simulink library "GRC_Lib"  (R2017b)
settings: Solver=VariableStepAuto  StartTime=0.0  StopTime=10.0  RelTol=1e-3  EnableMultiTasking=on
StartFcn:
  | set_param('AdvancedOperations','ZoomFactor','100');
undefined symbols (not defined in the file): Test
libraries: GRC_Lib x203, simulink x1
(part 3 of 4)

== system GRC_Lib/Routing ==
  Selector : Subsystem  TreatAsAtomicUnit=on  mask{IpDT=double, SizeUMsk=6}
      mask prompts: IpDT "Input U Data Type"; SizeUMsk "Input Port Size (Min 1)"
      mask init:
      | if isequal(str2num(get_param(gcb,'SizeUMsk')),[])
      |    if SizeUMsk<1
      |        error('*** ERROR ***    Input Port Size must be integer and >=1.');
      |    elseif SizeUMsk<256
      |        SizeU = SizeUMsk; 
      |        set_param([gcb '/Constant'],'OutDataTypeStr','uint8');
      |        set_param([gcb '/Constant'],'Value', mat2str(SizeUMsk-1));
      |    elseif SizeUMsk<=65535 
      |        SizeU = SizeUMsk; 
      |        set_param([gcb '/Constant'],'OutDataTypeStr','uint16');
      |        set_param([gcb '/Constant'],'Value', mat2str(SizeUMsk-1));
      |    else
      |        SizeU = SizeUMsk;
      |        set_param([gcb '/Constant'],'OutDataTypeStr','uint32');
      |        set_param([gcb '/Constant'],'Value', mat2str(SizeUMsk-1));
      |    end
      | else
      |     SizeNmbr = str2num(get_param(gcb,'SizeUMsk'));
      |    if SizeNmbr<1
      |        error('*** ERROR ***    Input Port Size must be integer and >=1.');
      |    elseif SizeNmbr<256
      |        SizeU = SizeUMsk;
      |        set_param([gcb '/Constant'],'OutDataTypeStr','uint8');
      |        set_param([gcb '/Constant'],'Value', mat2str(SizeNmbr-1));
      |    elseif SizeNmbr<=65535 
      |        SizeU = SizeNmbr;
      |        set_param([gcb '/Constant'],'OutDataTypeStr','uint16');
      |        set_param([gcb '/Constant'],'Value', mat2str(SizeNmbr-1));
      |    else
      |        SizeU = SizeNmbr;
      |        set_param([gcb '/Constant'],'OutDataTypeStr','uint32');
      |        set_param([gcb '/Constant'],'Value', mat2str(SizeNmbr-1));
      |    end 
      | end
      | 
      | DTStry = get_param(gcb,'IpDT');
      | try
      |     if isequal(DTStry,'boolean')
      |         FColor = '[0.901961, 0.313725, 0.078431]'; 
      |     elseif isequal(DTStry,'double')||isequal(DTStry,'single')
      |         FColor = '[0.313725, 0.117647, 0.352941]';  
      |     else
      |         FColor = '[0.196078, 0.549020, 0.549020]';
      |     end        
      | catch
      | end
      | set_param([gcb '/Y'],'ForegroundColor',FColor);
      | set_param(gcb,'ForegroundColor',FColor);
      settings: AttributesFormatString=SizeU = %<SizeUMsk>
      mask Callback SizeUMsk:
      | % if isequal(str2num(get_param(gcb,'SizeUMsk')),[])
      | %    if SizeUMsk<1
      | %        error('*** ERROR ***    Input Port Size must be integer and >=1.');
      | %    else
      | %    end
      | % else
      | %    if str2num(get_param(gcb,'SizeUMsk'))<1
      | %        error('*** ERROR ***    Input Port Size must be integer and >=1.');
      | %    else
      | %    end
      | % end
      mask Display:
      | % color('blue');
      | % disp('\bfSlctr','texmode','on');
      | image(imread('Selector.jpg'),[0.3,0.4,0.55,0.8]);
  Vbi_OilTempSensor : Subsystem  TreatAsAtomicUnit=on  mask(MessurementVaraibale){VariableName=Vbi_OilTempSensor, VariableType=Inherit: auto, S_Min=0, S_Max=100}
      mask prompts: VariableName "SignalName"; VariableType "VarableType"; S_Min "Min"; S_Max "Max"
      mask help: messurement Variable
      mask init:
      | hld = get_param([gcb '/In1'],'Object');
      | set(hld,'OutDataTypeStr',get_param(gcb,'VariableType'));
      | set(hld,'OutMin',get_param(gcb,'S_Min'));
      | set(hld,'OutMax',get_param(gcb,'S_Max'));
      | 
      | p_in1 =get_param([gcb '/In1'],'PortHandles');
      | hl_line = get_param(p_in1.Outport,'line');
      | set(hl_line,'Name',get_param(gcb,'VariableName'));
      | set(hl_line,'SignalObjectPackage','AUTOSAR4');
      | set(hl_line,'StorageClass','SimulinkGlobal');
      | 
      | DTStry = get_param(gcb,'VariableType');
      | try
      |     if isequal(DTStry,'boolean')
      |         FColor = '[0.901961, 0.313725, 0.078431]'; 
      |     elseif isequal(DTStry,'double')||isequal(DTStry,'single')
      |         FColor = '[0.313725, 0.117647, 0.352941]';  
      |     else
      |         FColor = '[0.196078, 0.549020, 0.549020]';
      |     end        
      | catch
      | end
      | set_param([gcb '/Out1'],'ForegroundColor',FColor);
      | set_param(gcb,'ForegroundColor',FColor);
      settings: RTWSystemCode=Inline
      mask Display:
      | %plot([0 .78 1 .78 0 0],[0 0 0.5 1 1 0]);
      | %plot([.78 .78],[0 1]);
      | %patch([0 .12 .12 0 0],[0 0 1 1 0],[0 0 0]);
      | color('black');
      | msk_block_name = get_param(gcb,'VariableName');
      | set_param(gcb,'Name',msk_block_name);
      | disp(get_param(gcb,'VariableName'));
      | %mp_in1 = find_system(gcb,'FindAll','on','type','line','name','label');
      | %mp_obj = get_param(mp_in1,'Object');
      | %set(mp_obj,'name',msk_block_name);
      | %set(mp_obj,'RTWStorageClass','SimulinkGloable');

== system GRC_Lib/SignalAttributes ==
  DTC : Subsystem  mask{OpDT=double}
      mask prompts: OpDT "Output Data Type"
      mask init:
      | set_param([gcb '/DTC'],'OutDataTypeStr',OpDT);
      | % set_param([gcb '/Odt'],'OutDataTypeStr',OpDT);
      | 
      | DTStry = get_param([gcb '/DTC'],'OutDataTypeStr');
      | try
      |     if isequal(DTStry,'boolean')
      |         FColor = '[0.901961, 0.313725, 0.078431]'; 
      |     elseif isequal(DTStry,'double')||isequal(DTStry,'single')
      |         FColor = '[0.313725, 0.117647, 0.352941]';  
      |     else
      |         FColor = '[0.196078, 0.549020, 0.549020]';
      |     end        
      | catch
      | end
      | set_param([gcb '/Odt'],'ForegroundColor',FColor);
      | set_param(gcb,'ForegroundColor',FColor);
      mask Display:
      | color('green');
      | disp(get_param(gcb,'OpDT'),'texmode','on');

== system GRC_Lib/SignalSwitch ==
  SWT2 : Subsystem  mask{OpDT=double}
      mask prompts: OpDT "Output Data Type"
      mask init:
      | DTStr = get_param(gcb,'OpDT');
      | try
      |     if isequal(DTStr,'boolean')
      |         FColor = '[0.901961, 0.313725, 0.078431]'; 
      |     elseif isequal(DTStr,'double')||isequal(DTStr,'single')
      |         FColor = '[0.313725, 0.117647, 0.352941]';  
      |     else
      |         FColor = '[0.196078, 0.549020, 0.549020]';
      |     end
      | catch
      | end
      | set_param([gcb '/T'],'ForegroundColor',FColor);
      | set_param([gcb '/F'],'ForegroundColor',FColor);
      | set_param([gcb '/y'],'ForegroundColor',FColor);
      mask Display:
      | % image('SwitchNN2.jpg');
      | image(imread('SWT2.jpg'),[0.25,0.15,0.55,0.85]);
  SWT3 : Subsystem  TreatAsAtomicUnit=on
      mask help:
      | if Rst = 1
      |    y = RstV;
      | else
      |     if E = 1
      |        y = u;
      |     else
      |        y = Z-1;
      |     end
      | end
      mask Display:
      | % color('red');
      | % disp('\bfSWT3','texmode','on');
      | image(imread('SWT3.jpg'),[0.3,0.1,0.55,0.95]);
  SWTM : Subsystem  mask{OpDT=double, DPOdr=Zero-based contiguous, NmbrIP=2, DPIdc={1,2,[3,4,5],6,7,[8,9,10],[11,12,13],14,15}, DPdft=Additional data port, cnt=0, b={}}
      mask prompts: OpDT "Output DataType"; DPOdr "Data port order"; NmbrIP "Number of data ports"; DPIdc "Data port indices (e.g. {1,[2,3]})"; DPdft "Data port for default case"
      mask init:
      | set_param([gcb '/S'],'Position',[195,123,225,137]);
      | set_param([gcb '/SWT'],'Position',[290,139,320,171]);
      | set_param([gcb '/y'],'Position',[385,148,415,162]);
      | 
      | %%%%%%%%%%%%%%%%%%%%%%%%%%%%%%%%%%%%%%%%%%%%%%%%%%%%%%%%%%%%%%%%%%%%%%%%%%%%%%%%%%%%%%%%%%%%%%%%%%%%%%%%%%%%%%%%%%%%%%%%
      | if isequal(get_param(gcb,'DPOdr'),'Zero-based contiguous')||isequal(get_param(gcb,'DPOdr'),'One-based contiguous')
      |    set_param(gcb,'MaskEnableString','on,on,on,off,off,off,off');
      |    set_param(gcb,'MaskVisibilityString','on,on,on,off,on,off,off');
      |    %%% Input port number detection  
      |    if isequal(str2num(get_param(gcb,'NmbrIP')),[])
      |       if NmbrIP<2
      |          error('*** ERROR_11 ***    Number of Input Port must be an Integer and >2.');
      |       else
      |       end
      |    else
      |       LocNmr = str2num(get_param(gcb,'NmbrIP'));
      |       if LocNmr<2
      |          error('*** ERROR_21 ***    Number of Input Port must be an Integer and >2.');
      |       else
      |       end
      |    end 
      |    
      |    LocVal = get_param(gcb,'NmbrIP');
      |    PortNmr = str2num(LocVal)+1;
      |     %%%%%%%%%%%%%%%%%%%%%%%%%%%%%%
      |     ExPtNmbr = length(get_param(gcb,'Blocks'))-4;
      |     if str2num(LocVal)<ExPtNmbr
      |        delete_line(gcb,'dft/1',['SWT/' mat2str(ExPtNmbr+2)]);%%% Delete existing Input lines
      |        dlte_block = strcat(gcb,'/dft');
      |        delete_block(dlte_block);   
      |        for i = PortNmr:ExPtNmbr
      |            delete_line(gcb, ['C' int2str(i) '/1'], ['SWT/' int2str(i+1)]);%%% Delete existing Input lines
      |            dlte_block = strcat(gcb,'/',['C' int2str(i)]);
      |            delete_block(dlte_block);
      |        end
      |     set_param([gcb '/SWT'],'Inputs',get_param(gcb,'NmbrIP')); %%%%%%%%%%%%%%%%%% TAKE CARE of the handles definition order !!!
      |     set_param([gcb '/SWT'],'DataPortOrder',get_param(gcb,'DPOdr')); %%%%%%%%%%%%%%%%%% TAKE CARE of the handles definition order !!!
      |     add_block('simulink/Sources/In1',[gcb '/dft']);
      |     set_param([gcb '/dft'],'Position',[195 123+50*PortNmr 225 137+50*PortNmr]);
      |     set_param([gcb '/SWT'],'Position',[290,139,320,171+20*PortNmr]);
      |     add_line(gcb,'dft/1',['SWT/' mat2str(PortNmr+1)]);
      |     %%% ***!=NOTE=!***  'DataPortOrder' handle definition should behind the 'Inputs' handle and 'DataPortIndices' handle definition.
      |     %%% ***!=NOTE=!*** Inorder to prevent time delay caused by middle variable, the set_param() had better capture data from get_param() function. 
      |     %%% Because some handles execute based on other handles existed value, and if the working handles running first, they will use relative handles' last time value or initial value for first step.
      |     elseif str2num(LocVal)>ExPtNmbr 
      |        delete_line(gcb,'dft/1',['SWT/' mat2str(ExPtNmbr+2)]);%%% Delete existing Input lines
      |        dlte_block = strcat(gcb,'/dft');
      |        delete_block(dlte_block);
      |        set_param([gcb '/SWT'],'Inputs',get_param(gcb,'NmbrIP')); %%%%%%%%%%%%%%%%%% TAKE CARE of the handles definition order !!!
      |        set_param([gcb '/SWT'],'DataPortOrder',get_param(gcb,'DPOdr')); %%%%%%%%%%%%%%%%%% TAKE CARE of the handles definition order !!!
      |        for j = (ExPtNmbr+1):str2num(LocVal)
      |             add_block('simulink/Sources/In1',[gcb '/C' int2str(j)]);
      |             set_param([gcb '/C' int2str(j)],'Position',[195 123+50*j 225 137+50*j]);
      |             add_line(gcb,['C' int2str(j) '/1'],['SWT/' int2str(j+1)]);
      |        end
      |        add_block('simulink/Sources/In1',[gcb '/dft']);
      |        set_param([gcb '/dft'],'Position',[195 123+50*PortNmr 225 137+50*PortNmr]);
      |        set_param([gcb '/SWT'],'Position',[290,139,320,171+20*PortNmr]);
      |        add_line(gcb,'dft/1',['SWT/' mat2str(PortNmr+1)]);
      |     else  
      |        set_param([gcb '/SWT'],'Inputs',get_param(gcb,'NmbrIP')); %%%%%%%%%%%%%%%%%% TAKE CARE of the handles definition order !!!
      |        set_param([gcb '/SWT'],'DataPortOrder',get_param(gcb,'DPOdr')); %%%%%%%%%%%%%%%%%% TAKE CARE of the handles definition order !!!
      |     end
      |     %%%%%%%%%%%%%%%%%%%%%%%%%%%%%%%            
      | else
      |     set_param(gcb,'MaskEnableString','on,on,off,on,off,off,off');
      |     set_param(gcb,'MaskVisibilityString','on,on,off,on,on,on,off');
      |     %%% Input Port number calculate
      |     Str = get_param(gcb,'DPIdc'); %Input string. ie. '{1,5,[2,3],4,[6,8],[10,30,40],11,60,7}'.
      |     DelimPosStr = strfind(Str,','); % Find out the ',' Position. ie.[3,5,8,11,13,16,19,23,26,30,33,36].
      |     DelimPosNmr =  length(DelimPosStr); % Calculate the ',' Number. ie. 12.
      |     RngStrLgr = strfind(Str, ']'); % Findout the ], position. ie. [10,18,29].
      |     CellNmr = length(RngStrLgr);    % Number of []. ie.3.
      |     RngStrSmr = strfind(Str, '['); % Findout the ,[ position. ie. [6,14,20]
      |     Cntr = 0;
      |     for m = 1:CellNmr
      |         for k = 1:DelimPosNmr
      |             if DelimPosStr(k)>RngStrSmr(m) && DelimPosStr(k)<RngStrLgr(m)
      |                Cntr = Cntr+1; % Calculate the'total ',' number between '[]', the ',' are useless for the statistic of total port number. 
      |             else
      |             end
      |         end
      |     end
      |     
      |     LocVal = mat2str(DelimPosNmr + 1 - Cntr); % Statistic of total port number. ie 12+1-4 = 9.
      |     PortNmr = str2num(LocVal)+1;
      |     %%%%%%%%%%%%%%%%%%%%%%%%%%%%%%
      |     ExPtNmbr = length(get_param(gcb,'Blocks'))-4;
      |     if str2num(LocVal)<ExPtNmbr
      |        delete_line(gcb,'dft/1',['SWT/' mat2str(ExPtNmbr+2)]);%%% Delete existing Input lines
      |        dlte_block = strcat(gcb,'/dft');
      |        delete_block(dlte_block);   
      |        for i = PortNmr:ExPtNmbr
      |            delete_line(gcb, ['C' int2str(i) '/1'], ['SWT/' int2str(i+1)]);%%% Delete existing Input lines
      |            dlte_block = strcat(gcb,'/',['C' int2str(i)]);
      |            delete_block(dlte_block);
      |        end
      |        set_param([gcb '/SWT'],'DataPortIndices',get_param(gcb,'DPIdc')); %%%%%%%%%%%%%%%%%% TAKE CARE of the handles definition order !!!
      |        set_param([gcb '/SWT'],'DataPortOrder',get_param(gcb,'DPOdr')); %%%%%%%%%%%%%%%%%% TAKE CARE of the handles definition order !!!
      |        add_block('simulink/Sources/In1',[gcb '/dft']);
      |        set_param([gcb '/dft'],'Position',[195 123+50*PortNmr 225 137+50*PortNmr]);
      |        set_param([gcb '/SWT'],'Position',[290,139,350,171+20*PortNmr]);
      |        add_line(gcb,'dft/1',['SWT/' mat2str(PortNmr+1)]);
      |     %%%%%%%% ***!=NOTE=!***  'DataPortOrder' handle definition should behind the 'Inputs' handle and 'DataPortIndices' handle definition.
      |     %%% Because some handles execute based on other handles existed value, and if the working handles running first, they will use relative handles' last time value or initial value for first step.
      |     elseif str2num(LocVal)>ExPtNmbr 
      |        delete_line(gcb,'dft/1',['SWT/' mat2str(ExPtNmbr+2)]);%%% Delete existing Input lines
      |        dlte_block = strcat(gcb,'/dft');
      |        delete_block(dlte_block);
      |        set_param([gcb '/SWT'],'DataPortIndices',get_param(gcb,'DPIdc')); %%%%%%%%%%%%%%%%%% TAKE CARE of the handles definition order !!!
      |        set_param([gcb '/SWT'],'DataPortOrder',get_param(gcb,'DPOdr')); %%%%%%%%%%%%%%%%%% TAKE CARE of the handles definition order !!!
      |        for j = (ExPtNmbr+1):str2num(LocVal)
      |             add_block('simulink/Sources/In1',[gcb '/C' int2str(j)]);
      |             set_param([gcb '/C' int2str(j)],'Position',[195 123+50*j 225 137+50*j]);
      |             add_line(gcb,['C' int2str(j) '/1'],['SWT/' int2str(j+1)]);
      |        end
      |        add_block('simulink/Sources/In1',[gcb '/dft']);
      |        set_param([gcb '/dft'],'Position',[195 123+50*PortNmr 225 137+50*PortNmr]);
      |        set_param([gcb '/SWT'],'Position',[290,139,350,171+20*PortNmr]);
      |        add_line(gcb,'dft/1',['SWT/' mat2str(PortNmr+1)]);
      |     else 
      |        set_param([gcb '/SWT'],'DataPortIndices',get_param(gcb,'DPIdc')); %%%%%%%%%%%%%%%%%% TAKE CARE of the handles definition order !!!
      |        set_param([gcb '/SWT'],'DataPortOrder',get_param(gcb,'DPOdr')); %%%%%%%%%%%%%%%%%% TAKE CARE of the handles definition order !!!
      |     end
      |     %%%%%%%%%%%%%%%%%%%%%%%%%%%%%%%
      | end
      | %%%%%%%%%%%%%%%%%%%%%%%%%%%%%%%%%%%%%%%%%%%%%%%%%%%%%%%%%%%%%%%%%%%%%%%%%%%%%%%%%%%%%%%%%%%%%%%%%%%%%%%%%%%%%%%%%%%%%
      | %%% Color setting
      | DTStr = get_param(gcb,'OpDT');
      | try
      |     if isequal(DTStr,'boolean')
      |         FColor = '[0.901961, 0.313725, 0.078431]'; 
      |     elseif isequal(DTStr,'double')||isequal(DTStr,'single')
      |         FColor = '[0.313725, 0.117647, 0.352941]';  
      |     else
      |         FColor = '[0.196078, 0.549020, 0.549020]';
      |     end        
      | catch
      | end
      | set_param([gcb '/SWT'],'OutDataTypeStr',DTStr);
      | set_param([gcb '/y'],'ForegroundColor',FColor);
      | 
      | 
      | %%%%%%%%%%%%%%%%%%%%%%%%%%%%%%%%%%%%%%%%%%%%%%%%%%%%%%%%%%%%%%%%%%%%%%%%%%%%%%%%%%%%%%%%%%%%%%%%%%5
      | if isequal(get_param(gcb,'DPOdr'),'Specify indices')
      | a = get_param(gcb,'DPIdc');
      | cnt = 1;
      | beginIndex = 1;
      | stopIndex  = 0;
      | oneArrayFlag = 0;
      | oneArrayFlagPre = 0;
      | beginIndexFlagPre = 0;
      | beginIndexFlag = 0;
      | cnt1stindex = 0;
      | symbolCnt = 0;
      | symbolIndexPre = 0;
      | for i = 1:length(a)
      |     if isequal(a(i), '[')
      |         oneArrayFlag = 1;
      |         beginIndex = i;
      |         continue;
      |     end
      |     if oneArrayFlag == 1
      |         symbolCnt = symbolCnt + 1;
      |         getDataSts = 0;
      |         symbolIndexPre = 0;
      |         if oneArrayFlagPre ~= oneArrayFlag
      |             oneArrayFlagPre = oneArrayFlag;
      |         end
      |         if isequal(a(i), ']')
      |             stopIndex = i;
      |             oneArrayFlag = 0;
      |             oneArrayFlagPre = 0;
      |             b{cnt} = a(beginIndex:stopIndex);
      |             cnt = cnt + 1;
      |             beginIndex = i+1;
      |         end
      |     end
      |     if isequal(a(i), '{')
      |         cnt1stindex = 1;
      |         beginIndex = 2;
      |         continue;
      |     end
      |     if oneArrayFlag ~= 1
      |         beginIndexFlag = 1;
      |         if ((beginIndexFlag ~= beginIndexFlagPre))
      |             beginIndex = i;
      |             beginIndexFlagPre = beginIndexFlag;
      |         end
      |         if isequal(a(i), ',')
      |             symbolCnt = symbolCnt + 1;
      |             symbolIndex = i;
      |             if symbolCnt == 1
      |                 b{cnt} = a(2:i-1);
      |                 cnt = cnt + 1;
      |                 beginIndexFlagPre = 0;
      |                 symbolIndexPre = symbolIndex;
      |                 continue;
      |             end           
      |             if symbolIndexPre ~= 0
      |                 b{cnt} = a(symbolIndexPre+1:symbolIndex-1);
      |                 cnt = cnt + 1;
      |             end
      |             symbolIndexPre = symbolIndex;
      |         end
      |     end
      | end
      | if i == length(a)
      |     if symbolIndex > symbolIndexPre
      |         if symbolIndexPre == 0
      |             
      |         else
      |             b{cnt} = a(symbolIndex+1:length(a)-1);
      |         end
      |     else
      |         b{cnt} = a(symbolIndexPre+1:length(a)-1);
      |     end
      | end
      | end
      | % disp(b)
      | % nn = cnt
      mask TypeOptions DPOdr: Zero-based contiguous | One-based contiguous | Specify indices
      mask Callback DPOdr:
      | %%% Input parameter detection
      | if strcmp(get_param(gcb,'DPOdr'),'Zero-based contiguous')||strcmp(get_param(gcb,'DPOdr'),'One-based contiguous')
      |       set_param(gcb,'MaskEnableString','on,on,on,off,off,off,off');
      |       set_param(gcb,'MaskVisibilityString','on,on,on,off,on,off,off');
      | else
      |       set_param(gcb,'MaskEnableString','on,on,off,on,off,off,off');
      |       set_param(gcb,'MaskVisibilityString','on,on,off,on,on,on,off');
      | end
      mask Callback NmbrIP:
      | % %%% Input port number detection
      | % if isequal(str2num(get_param(gcb,'NmbrIP')),[])
      | %    error('*** ERROR *** \n   Input must be an Integer and >2, and can not be a %s.',class(get_param(gcb,'NmbrIP')));
      | % elseif str2num(get_param(gcb,'NmbrIP'))<2
      | %    error('*** ERROR *** \n   Input must be an Integer and >2, and can not be a %s.',class(get_param(gcb,'NmbrIP')));
      | % else
      | % end
      mask TypeOptions DPdft: Additional data port
      mask Display:
      | % image('SWTM.jpg');
      | % image(imread('SWTM.jpg'),[0.35,0.05,0.45,0.9]);
      | % port_label('output',1,'nn');
      | 
      | %%%%%%%%%%%%%%%%%%%%%%%%%%%%%%%%%%%%%%%%%%%%%%%%%%%%%%%%%%%%%%%%%%%%%%%%%%%%%%%%%%%%%%%%%%%%%%%%%%%%%%%%%%%%%%%%%%%%%%%%
      | port_label('input',1,'S');
      | port_label('output',1,'y');
      | 
      | if isequal(get_param(gcb,'DPOdr'),'Zero-based contiguous')||isequal(get_param(gcb,'DPOdr'),'One-based contiguous')
      |     LocVal = str2num(get_param(gcb,'NmbrIP'));
      |        if isequal(get_param(gcb,'DPOdr'),'Zero-based contiguous')
      |            for i = 0:(LocVal-1)
      |                port_label('input',(i+2),int2str(i));
      |            end
      |        else
      |            for i = 1:LocVal
      |                port_label('input',(i+1),int2str(i));
      |            end
      |        end
      |        port_label('input',(LocVal)+2,'dft');
      | 
      | else
      |     try
      |         for i = 1:cnt %str2num(LocVal)
      |             port_label('input',i+1,b{i});
      |         end
      |     catch
      |     end
      |     Str = get_param(gcb,'DPIdc');
      |     DelimPosStr = strfind(Str,'}');
      |     RngStrLgr = strfind(Str, ']'); % Findout the ], position. ie. [10,18,29].
      |     if (DelimPosStr - max(RngStrLgr))==1
      |        port_label('input',cnt+1,'dft');
      |     else
      |        port_label('input',cnt+2,'dft');
      |     end
      | end

== system GRC_Lib/Sinks ==
  note: // The subsystem Source is used for system mask,
      | please don't mismatch Color&OutputDataType.
      |
      | -- Orange: Boolen
      | -- Green: Interger
      | -- Purple: Folat
      |
      | @ GRC|ATESTEO RLN 2016/9/22
  Out1 : Outport  OutDataTypeStr=boolean
      settings: AttributesFormatString=%<OutDataTypeStr>
  Out2 : Outport  Port=2  OutDataTypeStr=int32
      settings: AttributesFormatString=%<OutDataTypeStr>
  Out3 : Outport  Port=3  OutDataTypeStr=double
      settings: AttributesFormatString=%<OutDataTypeStr>

== system GRC_Lib/Sources ==
  note: // The subsystem Source is used for system mask,
      | please don't mismatch Color&OutputDataType.
      |
      | -- Orange: Boolen
      |    'ForegroundColor' = '[0.901961, 0.313725, 0.078431]'
      | -- Green: Interger
      |    'ForegroundColor' = '[0.196078, 0.549020, 0.549020]'
      | -- Purple: Float
      |    'ForegroundColor' = '[0.313725, 0.117647, 0.352941]'
      |
      | @ GRC|ATESTEO RLN 2016/9/22
  In1 : Inport  OutDataTypeStr=boolean
      settings: AttributesFormatString=%<OutDataTypeStr>
  In2 : Inport  Port=2  OutDataTypeStr=int32
      settings: AttributesFormatString=%<OutDataTypeStr>
  In3 : Inport  Port=3  OutDataTypeStr=double
      settings: AttributesFormatString=%<OutDataTypeStr>
  Constant : Constant  OutDataTypeStr=boolean
      settings: AttributesFormatString=%<OutDataTypeStr>
  Constant1 : Constant  OutDataTypeStr=int32
      settings: AttributesFormatString=%<OutDataTypeStr>
  Constant2 : Constant  OutDataTypeStr=double
      settings: AttributesFormatString=%<OutDataTypeStr>

== system GRC_Lib/AdvancedOperations/1D_DynamicLookupTable ==
  x : Inport
      settings: AttributesFormatString=%<OutDataTypeStr>
  xData : Inport  Port=2
      settings: AttributesFormatString=%<OutDataTypeStr>
  yData : Inport  Port=3
      settings: AttributesFormatString=%<OutDataTypeStr>
  Dynamic1D : simulink/Lookup Tables/Lookup Table Dynamic  LookUpMeth=Use Input Nearest  OutDataType=fixdt('single')  OutScaling=[]  OutputDataTypeScalingMode=Specify via dialog  OutDataTypeStr=single  DoSatur=off
      settings: SourceProductName=Simulink
  y : Outport
      settings: AttributesFormatString=%<OutDataTypeStr>
  wires:
  x/1 -> Dynamic1D/1
  xData/1 -> Dynamic1D/2
  yData/1 -> Dynamic1D/3
  Dynamic1D/1 -> y/1

== system GRC_Lib/AdvancedOperations/1D_LookupTableContrafunctional ==
  arrX : Inport
  arrY : Inport  Port=2
  y : Inport  Port=3
  Assertion : Assertion
  Chart : Stateflow chart  TreatAsAtomicUnit=on
  x : Outport
  err : Outport  Port=2
  wires:
  arrX/1 -> Chart/1(arrX)
  Chart/1(x) -> x/1
  arrY/1 -> Chart/2(arrY)
  y/1 -> Chart/3(y)
  Chart/2(err) -> Assertion/1, err/1

== system GRC_Lib/AdvancedOperations/2D_DynamicLookupTable ==
  x : Inport
      settings: AttributesFormatString=%<OutDataTypeStr>
  y : Inport  Port=2
      settings: AttributesFormatString=%<OutDataTypeStr>
  xData : Inport  Port=3
      settings: AttributesFormatString=%<OutDataTypeStr>
  yData : Inport  Port=4
      settings: AttributesFormatString=%<OutDataTypeStr>
  mData : Inport  Port=5
      settings: AttributesFormatString=%<OutDataTypeStr>
  Dynamic2D : Interpolation_n-D  TableSource=Input port  ExtrapMethod=Clip  RemoveProtectionIndex=on  OutDataTypeStr=double  RndMeth=Zero  IntermediateResultsDataTypeStr=double
      settings: InputPortMap=u0,u1,u2,u3,p2
  PrelookupX : PreLookup  BreakpointsDataSource=Input port  BreakpointsData=[10:10:110]  BeginIndexSearchUsingPreviousIndexResult=on  IndexDataTypeStr=uint8  RndMeth=Zero
      settings: InputPortMap=u0,p1
  PrelookupY : PreLookup  BreakpointsDataSource=Input port  BreakpointsData=[10:10:110]  BeginIndexSearchUsingPreviousIndexResult=on  IndexDataTypeStr=uint8  RndMeth=Zero
      settings: InputPortMap=u0,p1
  out : Outport
      settings: AttributesFormatString=%<OutDataTypeStr>
  wires:
  mData/1 -> Dynamic2D/5
  yData/1 -> PrelookupY/2
  y/1 -> PrelookupY/1
  xData/1 -> PrelookupX/2
  x/1 -> PrelookupX/1
  PrelookupY/2 -> Dynamic2D/4
  PrelookupY/1 -> Dynamic2D/3
  PrelookupX/2 -> Dynamic2D/2
  PrelookupX/1 -> Dynamic2D/1
  Dynamic2D/1 -> out/1

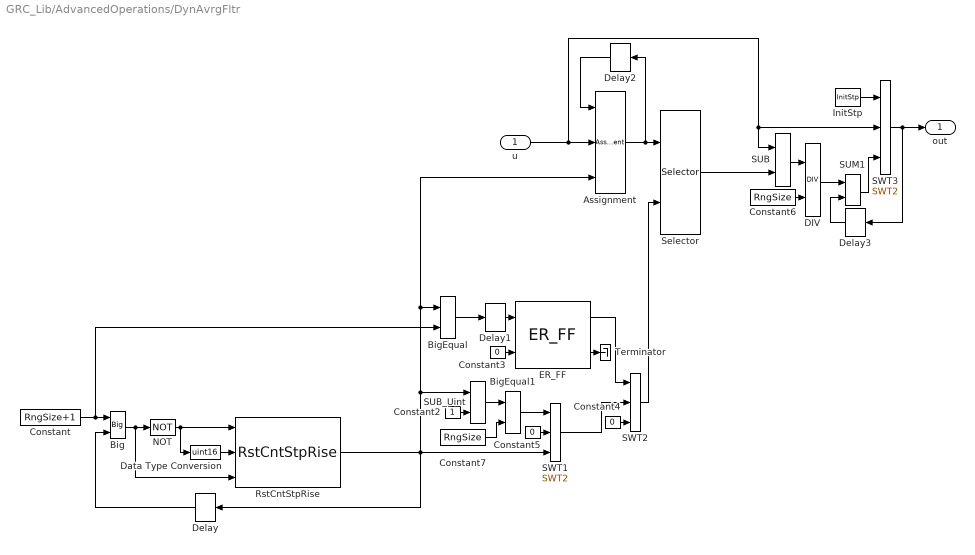
== system GRC_Lib/AdvancedOperations/DynAvrgFltr ==
  u : Inport
      settings: AttributesFormatString=%<OutDataTypeStr>
  Assignment : Assignment  DiagnosticForDimensions=Warning  IndexOptions=Index vector (port)  Indices=1  OutputSizes=1
  Big : GRC_Lib/ComparationOperation/Big  IpDT=double
  BigEqual : GRC_Lib/ComparationOperation/BigEqual  IpDT=double
  BigEqual1 : GRC_Lib/ComparationOperation/BigEqual  IpDT=double
  Constant : Constant  Value=RngSize+1  OutDataTypeStr=uint16
      settings: AttributesFormatString=%<OutDataTypeStr>
  Constant2 : Constant  OutDataTypeStr=uint16
  Constant3 : Constant  Value=0  OutDataTypeStr=boolean
  Constant4 : Constant  Value=0  OutDataTypeStr=uint16
  Constant5 : Constant  Value=0  OutDataTypeStr=uint16
  Constant6 : Constant  Value=RngSize  OutDataTypeStr=single
      settings: AttributesFormatString=%<OutDataTypeStr>
  Constant7 : Constant  Value=RngSize  OutDataTypeStr=uint16
  DIV : GRC_Lib/ArithmeticOperations/DIV  MinDivVal=1e-15  IpDT=single
  Data Type Conversion : DataTypeConversion  OutDataTypeStr=uint16
  Delay : GRC_Lib/Delay/Delay  IniV=0  IpDT=double
      settings: AttributesFormatString=%<IniV>
  Delay1 : GRC_Lib/Delay/Delay  IniV=0  IpDT=double
      settings: AttributesFormatString=%<IniV>
  Delay2 : GRC_Lib/Delay/Delay  IniV=zeros(1,(RngSize+1))  IpDT=double
      settings: AttributesFormatString=%<IniV>
  Delay3 : GRC_Lib/Delay/Delay  IniV=0  IpDT=double
      settings: AttributesFormatString=%<IniV>
  ER_FF : GRC_Lib/Memory/ER_FF  FalseVal=0  TrueVal=1
  InitStp : GRC_Lib/Delay/InitStp  OpDT_B=on  StpTp=~0 to 0  InitV=1  FnlV=5
  NOT : GRC_Lib/LogicalOperation/NOT
  RstCntStpRise : GRC_Lib/Counter_Timer/RstCntStpRise  IpDT=uint16
  SUB : GRC_Lib/ArithmeticOperations/SUB  IpDT=single  OFChk=on
  SUB_Uint : GRC_Lib/ArithmeticOperations/SUB_Uint  IpDT=uint16
  SUM1 : GRC_Lib/ArithmeticOperations/SUM  IpDT=single  OFChk=on
  SWT1 : GRC_Lib/SignalSwitch/SWT2  OpDT=double
  SWT2 : GRC_Lib/SignalSwitch/SWT2  OpDT=double
  SWT3 : GRC_Lib/SignalSwitch/SWT2  OpDT=double
  Selector : GRC_Lib/Routing/Selector  IpDT=double  SizeUMsk=RngSize+1
  Terminator : Terminator
  out : Outport
      settings: AttributesFormatString=%<OutDataTypeStr>
  wires:
  Constant/1 -> BigEqual/2, Big/1
  Big/1 -> RstCntStpRise/3, NOT/1
  NOT/1 -> Data Type Conversion/1, RstCntStpRise/1
  Delay/1 -> Big/2
  RstCntStpRise/1 -> Delay/1, SWT1/3, BigEqual/1, Assignment/3, SUB_Uint/1
  BigEqual/1 -> Delay1/1
  Delay1/1 -> ER_FF/1
  Constant3/1 -> ER_FF/2
  ER_FF/2 -> Terminator/1
  ER_FF/1 -> SWT2/1
  SWT1/1 -> SWT2/2
  Constant4/1 -> SWT2/3
  Constant5/1 -> SWT1/2
  u/1 -> SUB/1, SWT3/2, Assignment/2
  Delay2/1 -> Assignment/1
  Assignment/1 -> Delay2/1, Selector/1
  SWT2/1 -> Selector/2
  Selector/1 -> SUB/2
  SUB/1 -> DIV/1
  Constant6/1 -> DIV/2
  DIV/1 -> SUM1/1
  InitStp/1 -> SWT3/1
  SWT3/1 -> out/1, Delay3/1
  Delay3/1 -> SUM1/2
  SUM1/1 -> SWT3/3
  Data Type Conversion/1 -> RstCntStpRise/2
  Constant2/1 -> SUB_Uint/2
  SUB_Uint/1 -> BigEqual1/1
  Constant7/1 -> BigEqual1/2
  BigEqual1/1 -> SWT1/1

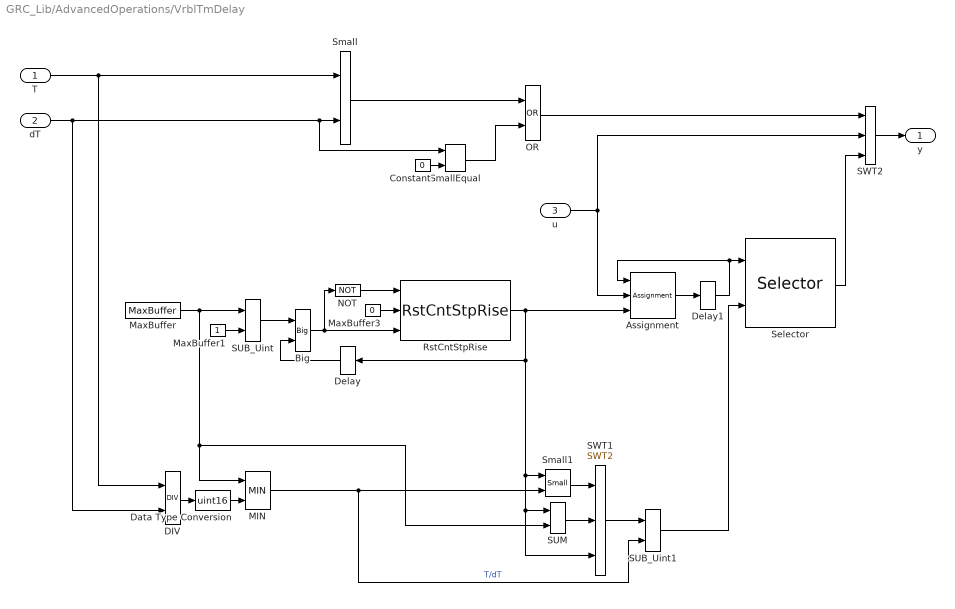
== system GRC_Lib/AdvancedOperations/VrblTmDelay ==
  T : Inport
      settings: AttributesFormatString=%<OutDataTypeStr>
  dT : Inport  Port=2
      settings: AttributesFormatString=%<OutDataTypeStr>
  u : Inport  Port=3
      settings: AttributesFormatString=%<OutDataTypeStr>
  Assignment : Assignment  IndexMode=Zero-based  DiagnosticForDimensions=Warning  IndexOptions=Index vector (port)  Indices=1  OutputSizes=1
  Big : GRC_Lib/ComparationOperation/Big  IpDT=double
  Constant : Constant  Value=0  OutDataTypeStr=double
      settings: AttributesFormatString=%<OutDataTypeStr>
  DIV : GRC_Lib/ArithmeticOperations/DIV  MinDivVal=1e-15  IpDT=double
      settings: AttributesFormatString=%<IpDT>
  Data Type Conversion : DataTypeConversion  OutDataTypeStr=uint16
  Delay : GRC_Lib/Delay/Delay  IniV=0  IpDT=double
  Delay1 : GRC_Lib/Delay/Delay  IniV=initValue*ones(1,MaxBuffer)  IpDT=double
  MIN : GRC_Lib/ComparationOperation/MIN  OpDT=double
  MaxBuffer : Constant  Value=MaxBuffer  OutDataTypeStr=uint16
  MaxBuffer1 : Constant  OutDataTypeStr=uint16
  MaxBuffer3 : Constant  Value=0  OutDataTypeStr=uint16
  NOT : GRC_Lib/LogicalOperation/NOT
  OR : GRC_Lib/LogicalOperation/OR  n=2
  RstCntStpRise : GRC_Lib/Counter_Timer/RstCntStpRise  IpDT=uint16
  SUB_Uint : GRC_Lib/ArithmeticOperations/SUB_Uint  IpDT=uint16
      settings: AttributesFormatString=|
      | SUB_Uint
      | %<IpDT>
  SUB_Uint1 : GRC_Lib/ArithmeticOperations/SUB_Uint  IpDT=uint16
      settings: AttributesFormatString=SUB_Uint
  SUM : GRC_Lib/ArithmeticOperations/SUM  IpDT=uint16  OFChk=off
  SWT1 : GRC_Lib/SignalSwitch/SWT2  OpDT=double
  SWT2 : GRC_Lib/SignalSwitch/SWT2  OpDT=double
  Selector : GRC_Lib/Routing/Selector  IpDT=double  SizeUMsk=1
  Small : GRC_Lib/ComparationOperation/Small  IpDT=double
  Small1 : GRC_Lib/ComparationOperation/Small  IpDT=double
  SmallEqual : GRC_Lib/ComparationOperation/SmallEqual  IpDT=double
  y : Outport
      settings: AttributesFormatString=%<OutDataTypeStr>
  wires:
  MaxBuffer1/1 -> SUB_Uint/2
  SUB_Uint/1 -> Big/1
  Big/1 -> NOT/1, RstCntStpRise/3
  NOT/1 -> RstCntStpRise/1
  MaxBuffer3/1 -> RstCntStpRise/2
  RstCntStpRise/1 -> SWT1/3, SUM/1, Small1/1, Delay/1, Assignment/3
  Delay/1 -> Big/2
  u/1 -> Assignment/2, SWT2/2
  Assignment/1 -> Delay1/1
  Delay1/1 -> Selector/1, Assignment/1
  SWT2/1 -> y/1
  T/1 -> Small/1, DIV/1
  dT/1 -> SmallEqual/1, Small/2, DIV/2
  OR/1 -> SWT2/1
  Small/1 -> OR/1
  Constant/1 -> SmallEqual/2
  SmallEqual/1 -> OR/2
  Selector/1 -> SWT2/3
  DIV/1 -> Data Type Conversion/1
  Data Type Conversion/1 -> MIN/2
  MIN/1 -> SUB_Uint1/2, Small1/2  "T/dT"
  Small1/1 -> SWT1/1
  SUM/1 -> SWT1/2
  SWT1/1 -> SUB_Uint1/1
  SUB_Uint1/1 -> Selector/2
  MaxBuffer/1 -> SUM/2, MIN/1, SUB_Uint/1

== system GRC_Lib/ArithmeticOperations/DIV ==
  In1 : Inport
      settings: AttributesFormatString=%<OutDataTypeStr>
  In2 : Inport  Port=2
      settings: AttributesFormatString=%<OutDataTypeStr>
  BigEqual : GRC_Lib/ComparationOperation/BigEqual  IpDT=int8
  Constant1 : Constant  Value=0  OutDataTypeStr=int8  SampleTime=-1
  Constant2 : Constant  Value=abs(MinVal)  OutDataTypeStr=double  SampleTime=-1
  Constant3 : Constant  Value=-abs(MinVal)  OutDataTypeStr=double  SampleTime=-1
  Divide : Product  Inputs=*/  OutDataTypeStr=int8  RndMeth=Zero
  MAX : GRC_Lib/ComparationOperation/MAX  OpDT=int8
  MIN : GRC_Lib/ComparationOperation/MIN  OpDT=int8
  SWT2 : GRC_Lib/SignalSwitch/SWT2  OpDT=double
  Out : Outport
      settings: AttributesFormatString=%<OutDataTypeStr>
  wires:
  Divide/1 -> Out/1
  In1/1 -> Divide/1
  SWT2/1 -> Divide/2
  MIN/1 -> SWT2/3
  MAX/1 -> SWT2/2
  BigEqual/1 -> SWT2/1
  Constant1/1 -> BigEqual/2
  Constant3/1 -> MIN/2
  Constant2/1 -> MAX/2
  In2/1 -> MAX/1, MIN/1, BigEqual/1

== system GRC_Lib/ArithmeticOperations/GAIN ==
  In1 : Inport
      settings: AttributesFormatString=%<OutDataTypeStr>
  Gain1 : Gain  Gain=GAIN  OutDataTypeStr=double
      settings: AttributesFormatString=%<OutDataTypeStr>
  Out1 : Outport
      settings: AttributesFormatString=%<OutDataTypeStr>
  wires:
  Gain1/1 -> Out1/1
  In1/1 -> Gain1/1

== system GRC_Lib/ArithmeticOperations/MUL ==
  In1 : Inport
      settings: AttributesFormatString=%<OutDataTypeStr>
  In2 : Inport  Port=2
      settings: AttributesFormatString=%<OutDataTypeStr>
  Mul1 : Product  OutDataTypeStr=double
      settings: AttributesFormatString=%<OutDataTypeStr>
  Out1 : Outport
      settings: AttributesFormatString=%<OutDataTypeStr>
  wires:
  In1/1 -> Mul1/1
  In2/1 -> Mul1/2
  Mul1/1 -> Out1/1

== system GRC_Lib/ArithmeticOperations/NEG ==
  In1 : Inport
      settings: AttributesFormatString=%<OutDataTypeStr>
  Neg1 : Gain  Gain=-1  OutDataTypeStr=double
      settings: AttributesFormatString=%<OutDataTypeStr>
  Out1 : Outport
      settings: AttributesFormatString=%<OutDataTypeStr>
  wires:
  Neg1/1 -> Out1/1
  In1/1 -> Neg1/1

== system GRC_Lib/ArithmeticOperations/SUB ==
  In1 : Inport
      settings: AttributesFormatString=%<OutDataTypeStr>
  In2 : Inport  Port=2
      settings: AttributesFormatString=%<OutDataTypeStr>
  Sub1 : Sum  Inputs=+-  OutDataTypeStr=double
      settings: AttributesFormatString=%<OutDataTypeStr>
  Out1 : Outport
      settings: AttributesFormatString=%<OutDataTypeStr>
  wires:
  In1/1 -> Sub1/1
  In2/1 -> Sub1/2
  Sub1/1 -> Out1/1

== system GRC_Lib/ArithmeticOperations/SUB_Uint ==
  In1 : Inport
      settings: AttributesFormatString=%<OutDataTypeStr>
  In2 : Inport  Port=2
      settings: AttributesFormatString=%<OutDataTypeStr>
  Constant : Constant  Value=0  OutDataTypeStr=uint8
  SWT2 : GRC_Lib/SignalSwitch/SWT2  OpDT=double
  Small : GRC_Lib/ComparationOperation/Small  IpDT=double
  Sub : Sum  Inputs=+-
  Out : Outport
      settings: AttributesFormatString=%<OutDataTypeStr>
  wires:
  Sub/1 -> SWT2/3
  SWT2/1 -> Out/1
  Constant/1 -> SWT2/2
  Small/1 -> SWT2/1
  In2/1 -> Sub/2, Small/2
  In1/1 -> Sub/1, Small/1

== system GRC_Lib/ArithmeticOperations/SUM ==
  In1 : Inport
      settings: AttributesFormatString=%<OutDataTypeStr>
  In2 : Inport  Port=2
      settings: AttributesFormatString=%<OutDataTypeStr>
  Sum1 : Sum  OutDataTypeStr=single
      settings: AttributesFormatString=%<OutDataTypeStr>
  Out1 : Outport
      settings: AttributesFormatString=%<OutDataTypeStr>
  wires:
  In1/1 -> Sum1/1
  In2/1 -> Sum1/2
  Sum1/1 -> Out1/1

== system GRC_Lib/BitOperations/AndBit_32bit ==
  In1 : Inport
      settings: AttributesFormatString=%<OutDataTypeStr>
  In2 : Inport  Port=2
      settings: AttributesFormatString=%<OutDataTypeStr>
  Chart : Stateflow chart  TreatAsAtomicUnit=on
  Out : Outport
      settings: AttributesFormatString=%<OutDataTypeStr>
  wires:
  In1/1 -> Chart/1(In1)
  In2/1 -> Chart/2(In2)
  Chart/1(Out) -> Out/1

== system GRC_Lib/BitOperations/BitAND ==
  In1 : Inport
      settings: AttributesFormatString=%<OutDataTypeStr>
  In2 : Inport  Port=2
      settings: AttributesFormatString=%<OutDataTypeStr>
  Chart : Stateflow chart  TreatAsAtomicUnit=on
  Out : Outport
      settings: AttributesFormatString=%<OutDataTypeStr>
  wires:
  Chart/1(Out) -> Out/1
  In2/1 -> Chart/2(In2)
  In1/1 -> Chart/1(In1)

== system GRC_Lib/BitOperations/BitClear_Filter ==
  u : Inport
      settings: AttributesFormatString=%<OutDataTypeStr>
  FltrV : Inport  Port=2
      settings: AttributesFormatString=%<OutDataTypeStr>
  Chart : Stateflow chart  TreatAsAtomicUnit=on
  y : Outport
      settings: AttributesFormatString=%<OutDataTypeStr>
  wires:
  u/1 -> Chart/1(In)
  FltrV/1 -> Chart/2(Fltr)
  Chart/1(Out) -> y/1

== system GRC_Lib/BitOperations/BitFltrDtct ==
  u : Inport
      settings: AttributesFormatString=%<OutDataTypeStr>
  Fltr : Inport  Port=2
      settings: AttributesFormatString=%<OutDataTypeStr>
  BitAND : GRC_Lib/BitOperations/BitAND  IpDT=uint32
  Equal : GRC_Lib/ComparationOperation/Equal  IpDT=double
  y : Outport
      settings: AttributesFormatString=%<OutDataTypeStr>
  wires:
  BitAND/1 -> Equal/1
  u/1 -> BitAND/1
  Fltr/1 -> Equal/2, BitAND/2
  Equal/1 -> y/1

== system GRC_Lib/BitOperations/BitOR ==
  In1 : Inport
      settings: AttributesFormatString=%<OutDataTypeStr>
  In2 : Inport  Port=2
      settings: AttributesFormatString=%<OutDataTypeStr>
  Chart : Stateflow chart  TreatAsAtomicUnit=on
  Out : Outport
      settings: AttributesFormatString=%<OutDataTypeStr>
  wires:
  Chart/1(Out) -> Out/1
  In2/1 -> Chart/2(In2)
  In1/1 -> Chart/1(In1)

== system GRC_Lib/BitOperations/BitXOR ==
  In1 : Inport
      settings: AttributesFormatString=%<OutDataTypeStr>
  In2 : Inport  Port=2
      settings: AttributesFormatString=%<OutDataTypeStr>
  Chart : Stateflow chart  TreatAsAtomicUnit=on
  Out : Outport
      settings: AttributesFormatString=%<OutDataTypeStr>
  wires:
  Chart/1(Out) -> Out/1
  In2/1 -> Chart/2(In2)
  In1/1 -> Chart/1(In1)

== system GRC_Lib/BitOperations/ClearBit_32bit ==
  u : Inport
      settings: AttributesFormatString=%<OutDataTypeStr>
  bit : Inport  Port=2
      settings: AttributesFormatString=%<OutDataTypeStr>
  Chart : Stateflow chart  TreatAsAtomicUnit=on
  One : Constant  OutDataTypeStr=uint32
      settings: AttributesFormatString=%<OutDataTypeStr>
  data_length : Constant  Value=dataLength  OutDataTypeStr=uint8
      settings: AttributesFormatString=%<OutDataTypeStr>
  msb_clear_flag : Constant  Value=msbClearFlag  OutDataTypeStr=uint32
      settings: AttributesFormatString=%<OutDataTypeStr>
  y : Outport
      settings: AttributesFormatString=%<OutDataTypeStr>
  wires:
  Chart/1(Out) -> y/1
  u/1 -> Chart/1(bitArray)
  bit/1 -> Chart/2(position)
  One/1 -> Chart/3(one)
  msb_clear_flag/1 -> Chart/4(msb_clear_flag)
  data_length/1 -> Chart/5(data_length)

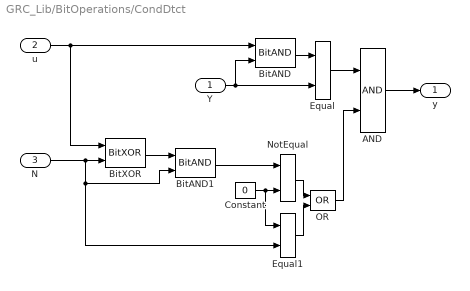
== system GRC_Lib/BitOperations/CondDtct ==
  Y : Inport
      settings: AttributesFormatString=%<OutDataTypeStr>
  u : Inport  Port=2
      settings: AttributesFormatString=%<OutDataTypeStr>
  N : Inport  Port=3
      settings: AttributesFormatString=%<OutDataTypeStr>
  AND : GRC_Lib/LogicalOperation/AND  n=2
  BitAND : GRC_Lib/BitOperations/BitAND  IpDT=uint8
  BitAND1 : GRC_Lib/BitOperations/BitAND  IpDT=uint8
  BitXOR : GRC_Lib/BitOperations/BitXOR  IpDT=uint8
  Constant : Constant  Value=0  OutDataTypeStr=boolean
  Equal : GRC_Lib/ComparationOperation/Equal  IpDT=double
  Equal1 : GRC_Lib/ComparationOperation/Equal  IpDT=double
  NotEqual : GRC_Lib/ComparationOperation/NotEqual  IpDT=double
  OR : GRC_Lib/LogicalOperation/OR  n=2
  y : Outport
      settings: AttributesFormatString=%<OutDataTypeStr>
  wires:
  u/1 -> BitXOR/1, BitAND/1
  BitAND/1 -> Equal/1
  Y/1 -> BitAND/2, Equal/2
  Equal/1 -> AND/1
  N/1 -> BitXOR/2, BitAND1/2, Equal1/2
  BitXOR/1 -> BitAND1/1
  BitAND1/1 -> NotEqual/1
  Constant/1 -> Equal1/1, NotEqual/2
  NotEqual/1 -> OR/1
  Equal1/1 -> OR/2
  OR/1 -> AND/2
  AND/1 -> y/1

== system GRC_Lib/BitOperations/GetBit_32bit ==
  u : Inport
      settings: AttributesFormatString=%<OutDataTypeStr>
  bit : Inport  Port=2
      settings: AttributesFormatString=%<OutDataTypeStr>
  Chart : Stateflow chart  TreatAsAtomicUnit=on
  data_length : Constant  Value=datalength  OutDataTypeStr=uint8
      settings: AttributesFormatString=%<OutDataTypeStr>
  y : Outport
      settings: AttributesFormatString=%<OutDataTypeStr>
  wires:
  Chart/1(BitValue) -> y/1
  u/1 -> Chart/1(Value)
  bit/1 -> Chart/2(BitPos)
  data_length/1 -> Chart/3(data_length)

== system GRC_Lib/BitOperations/MSB ==
  u : Inport
      settings: AttributesFormatString=%<OutDataTypeStr>
  Chart : Stateflow chart  TreatAsAtomicUnit=on
  Index : Constant  Value=IniIdx  OutDataTypeStr=int8
      settings: AttributesFormatString=%<OutDataTypeStr>
  RefBinary : Constant  Value=[2 12 240 65280 4294901760]  OutDataTypeStr=uint32
      settings: AttributesFormatString=%<OutDataTypeStr>
  RefPos : Constant  Value=[1 2 4 8 16]  OutDataTypeStr=uint8
      settings: AttributesFormatString=%<OutDataTypeStr>
  y : Outport
      settings: AttributesFormatString=%<OutDataTypeStr>
  wires:
  u/1 -> Chart/1(u)
  Index/1 -> Chart/2(i)
  RefBinary/1 -> Chart/3(RefBin)
  RefPos/1 -> Chart/4(RefPos)
  Chart/1(Pos) -> y/1

== system GRC_Lib/BitOperations/NOT ==
  In1 : Inport
      settings: AttributesFormatString=%<OutDataTypeStr>
  Chart : Stateflow chart  TreatAsAtomicUnit=on
  Out : Outport
      settings: AttributesFormatString=%<OutDataTypeStr>
  wires:
  Chart/1(Out) -> Out/1
  In1/1 -> Chart/1(In)

== system GRC_Lib/BitOperations/SetBit_32bit ==
  E : Inport
      settings: AttributesFormatString=%<OutDataTypeStr>
  u : Inport  Port=2
      settings: AttributesFormatString=%<OutDataTypeStr>
  bit : Inport  Port=3
      settings: AttributesFormatString=%<OutDataTypeStr>
  Chart : Stateflow chart  TreatAsAtomicUnit=on
  data_length : Constant  Value=datalength  OutDataTypeStr=uint8
      settings: AttributesFormatString=%<OutDataTypeStr>
  msb_set_flag : Constant  Value=msbSetFlag  OutDataTypeStr=uint32
      settings: AttributesFormatString=%<OutDataTypeStr>
  y : Outport
      settings: AttributesFormatString=%<OutDataTypeStr>
  wires:
  E/1 -> Chart/1(Enable)
  u/1 -> Chart/2(u)
  bit/1 -> Chart/3(BitPos)
  data_length/1 -> Chart/4(data_length)
  msb_set_flag/1 -> Chart/5(msb_set_flag)
  Chart/1(y) -> y/1

== system GRC_Lib/BitOperations/SetBit_Count ==
  u : Inport
      settings: AttributesFormatString=%<OutDataTypeStr>
  Chart : Stateflow chart  TreatAsAtomicUnit=on
  c : Outport
      settings: AttributesFormatString=%<OutDataTypeStr>
  wires:
  u/1 -> Chart/1(u)
  Chart/1(count) -> c/1

== system GRC_Lib/ComparationOperation/Big ==
  u1 : Inport
      settings: AttributesFormatString=%<OutDataTypeStr>
  u2 : Inport  Port=2
      settings: AttributesFormatString=%<OutDataTypeStr>
  Relational Operator : RelationalOperator  Operator=>  OutDataTypeStr=boolean  RndMeth=Nearest
  y : Outport
      settings: AttributesFormatString=%<OutDataTypeStr>
  wires:
  u1/1 -> Relational Operator/1
  u2/1 -> Relational Operator/2
  Relational Operator/1 -> y/1

== system GRC_Lib/ComparationOperation/BigEqual ==
  u1 : Inport
      settings: AttributesFormatString=%<OutDataTypeStr>
  u2 : Inport  Port=2
      settings: AttributesFormatString=%<OutDataTypeStr>
  Relational Operator : RelationalOperator  OutDataTypeStr=boolean  RndMeth=Nearest
  y : Outport
      settings: AttributesFormatString=%<OutDataTypeStr>
  wires:
  Relational Operator/1 -> y/1
  u2/1 -> Relational Operator/2
  u1/1 -> Relational Operator/1

== system GRC_Lib/ComparationOperation/Equal ==
  u1 : Inport
      settings: AttributesFormatString=%<OutDataTypeStr>
  u2 : Inport  Port=2
      settings: AttributesFormatString=%<OutDataTypeStr>
  Relational Operator : RelationalOperator  Operator===  OutDataTypeStr=boolean  RndMeth=Nearest
  y : Outport
      settings: AttributesFormatString=%<OutDataTypeStr>
  wires:
  u1/1 -> Relational Operator/1
  u2/1 -> Relational Operator/2
  Relational Operator/1 -> y/1

== system GRC_Lib/ComparationOperation/FltEqual ==
  u1 : Inport
      settings: AttributesFormatString=%<OutDataTypeStr>
  u2 : Inport  Port=2
      settings: AttributesFormatString=%<OutDataTypeStr>
  Abs : Abs
  Abs1 : Abs
  Abs2 : Abs
  Epslion : Constant  Value=err  OutDataTypeStr=single
  MIN : GRC_Lib/ComparationOperation/MIN  OpDT=single
  Product : Product
  Relational Operator : RelationalOperator  Operator=<=  OutDataTypeStr=boolean  RndMeth=Nearest
  Subtract : Sum  Inputs=+-
  y : Outport
      settings: AttributesFormatString=%<OutDataTypeStr>
  wires:
  u1/1 -> Abs1/1, Subtract/1
  u2/1 -> Abs2/1, Subtract/2
  Subtract/1 -> Abs/1
  Abs/1 -> Relational Operator/1
  Abs1/1 -> MIN/2
  Abs2/1 -> MIN/1
  MIN/1 -> Product/1
  Epslion/1 -> Product/2
  Product/1 -> Relational Operator/2
  Relational Operator/1 -> y/1

== system GRC_Lib/ComparationOperation/FltNotEqual ==
  u1 : Inport
      settings: AttributesFormatString=%<OutDataTypeStr>
  u2 : Inport  Port=2
      settings: AttributesFormatString=%<OutDataTypeStr>
  Abs : Abs
  Abs1 : Abs
  Abs2 : Abs
  Epslion : Constant  Value=err  OutDataTypeStr=double
  MIN : GRC_Lib/ComparationOperation/MIN  OpDT=double
  Product : Product
  Relational Operator : RelationalOperator  Operator=>  OutDataTypeStr=boolean  RndMeth=Nearest
  Subtract : Sum  Inputs=+-
  y : Outport
      settings: AttributesFormatString=%<OutDataTypeStr>
  wires:
  u1/1 -> Abs1/1, Subtract/1
  u2/1 -> Abs2/1, Subtract/2
  Subtract/1 -> Abs/1
  Abs/1 -> Relational Operator/1
  Abs1/1 -> MIN/2
  Abs2/1 -> MIN/1
  MIN/1 -> Product/1
  Epslion/1 -> Product/2
  Product/1 -> Relational Operator/2
  Relational Operator/1 -> y/1

== system GRC_Lib/ComparationOperation/MAX ==
  In1 : Inport
      settings: AttributesFormatString=%<OutDataTypeStr>
  In2 : Inport  Port=2
      settings: AttributesFormatString=%<OutDataTypeStr>
  SWT2 : GRC_Lib/SignalSwitch/SWT2  OpDT=int32
  Small : GRC_Lib/ComparationOperation/Small  IpDT=double
  Out : Outport
      settings: AttributesFormatString=%<OutDataTypeStr>
  wires:
  In1/1 -> Small/1, SWT2/3
  In2/1 -> Small/2, SWT2/2
  Small/1 -> SWT2/1
  SWT2/1 -> Out/1

== system GRC_Lib/ComparationOperation/MIN ==
  In1 : Inport
      settings: AttributesFormatString=%<OutDataTypeStr>
  In2 : Inport  Port=2
      settings: AttributesFormatString=%<OutDataTypeStr>
  Big : GRC_Lib/ComparationOperation/Big  IpDT=double
  SWT2 : GRC_Lib/SignalSwitch/SWT2  OpDT=double
  Out : Outport
      settings: AttributesFormatString=%<OutDataTypeStr>
  wires:
  In1/1 -> Big/1, SWT2/3
  In2/1 -> Big/2, SWT2/2
  Big/1 -> SWT2/1
  SWT2/1 -> Out/1

== system GRC_Lib/ComparationOperation/NotEqual ==
  u1 : Inport
      settings: AttributesFormatString=%<OutDataTypeStr>
  u2 : Inport  Port=2
      settings: AttributesFormatString=%<OutDataTypeStr>
  Relational Operator : RelationalOperator  Operator=~=  OutDataTypeStr=boolean  RndMeth=Nearest
  y : Outport
      settings: AttributesFormatString=%<OutDataTypeStr>
  wires:
  Relational Operator/1 -> y/1
  u2/1 -> Relational Operator/2
  u1/1 -> Relational Operator/1

== system GRC_Lib/ComparationOperation/Small ==
  u1 : Inport
      settings: AttributesFormatString=%<OutDataTypeStr>
  u2 : Inport  Port=2
      settings: AttributesFormatString=%<OutDataTypeStr>
  Relational Operator : RelationalOperator  Operator=<  OutDataTypeStr=boolean  RndMeth=Nearest
  y : Outport
      settings: AttributesFormatString=%<OutDataTypeStr>
  wires:
  Relational Operator/1 -> y/1
  u2/1 -> Relational Operator/2
  u1/1 -> Relational Operator/1

== system GRC_Lib/ComparationOperation/SmallEqual ==
  u1 : Inport
      settings: AttributesFormatString=%<OutDataTypeStr>
  u2 : Inport  Port=2
      settings: AttributesFormatString=%<OutDataTypeStr>
  Relational Operator : RelationalOperator  Operator=<=  OutDataTypeStr=boolean  RndMeth=Nearest
  y : Outport
      settings: AttributesFormatString=%<OutDataTypeStr>
  wires:
  u1/1 -> Relational Operator/1
  u2/1 -> Relational Operator/2
  Relational Operator/1 -> y/1

== system GRC_Lib/ComparationOperation/abu ==
  Max : Inport
      settings: AttributesFormatString=%<OutDataTypeStr>
  u : Inport  Port=2
      settings: AttributesFormatString=%<OutDataTypeStr>
  Min : Inport  Port=3
      settings: AttributesFormatString=%<OutDataTypeStr>
  Logical Operator : Logic  AllPortsSameDT=off  OutDataTypeStr=boolean
  Relational Operator : RelationalOperator  Operator=>  OutDataTypeStr=boolean  RndMeth=Nearest
  Relational Operator1 : RelationalOperator  OutDataTypeStr=boolean  RndMeth=Nearest
  y : Outport
      settings: AttributesFormatString=%<OutDataTypeStr>
  wires:
  Relational Operator/1 -> Logical Operator/1
  Relational Operator1/1 -> Logical Operator/2
  Logical Operator/1 -> y/1
  u/1 -> Relational Operator1/1, Relational Operator/2
  Max/1 -> Relational Operator/1
  Min/1 -> Relational Operator1/2
